simulink model "Isat"  (Simulink 7.5)
settings: Solver=ode45  StartTime=0.0  StopTime=10.0  RelTol=1e-3
settings Model: Creator=dell  LastModifiedBy=dell

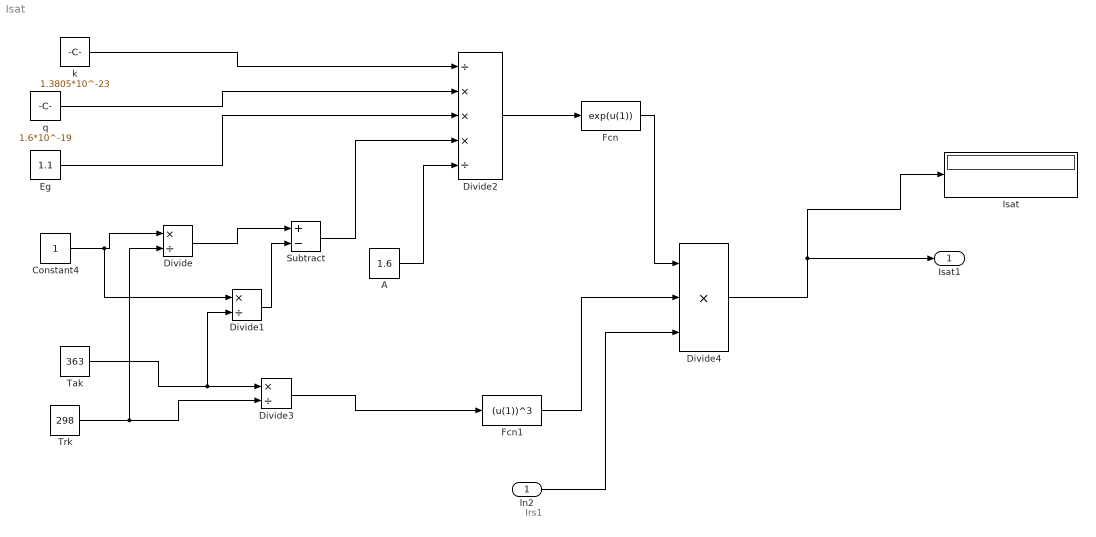
== system Isat ==
  note: Irs1
  In2 : Inport  OutDataType=fixdt(1, 16)  OutScaling=2^0
  A : Constant  Value=1.6  OutDataType=fixdt(1, 16)  OutScaling=2^0
  Constant4 : Constant  OutDataType=fixdt(1, 16)  OutScaling=2^0
  Divide : Product  Inputs=*/  OutDataType=fixdt(1, 16)  OutScaling=2^-10
  Divide1 : Product  Inputs=*/  OutDataType=fixdt(1, 16)  OutScaling=2^-10
  Divide2 : Product  Inputs=/***/  OutDataType=fixdt(1, 16)  OutScaling=2^-10
  Divide3 : Product  Inputs=*/  OutDataType=fixdt(1, 16)  OutScaling=2^-10
  Divide4 : Product  Inputs=***  OutDataType=fixdt(1, 16)  OutScaling=2^-10
  Eg : Constant  Value=1.1  OutDataType=fixdt(1, 16)  OutScaling=2^0
  Fcn : Fcn  Expr=exp(u(1))
  Fcn1 : Fcn  Expr=(u(1))^3
  Isat : Display
  Subtract : Sum  Inputs=+-  OutDataType=fixdt(1, 16)  OutScaling=2^-10
  Tak : Constant  Value=363  OutDataType=fixdt(1, 16)  OutScaling=2^0
  Trk : Constant  Value=298  OutDataType=fixdt(1, 16)  OutScaling=2^0
  k : Constant  Value=1.3805*10^-23  OutDataType=fixdt(1, 16)  OutScaling=2^0
  q : Constant  Value=1.6*10^-19  OutDataType=fixdt(1, 16)  OutScaling=2^0
  Isat1 : Outport  OutDataType=fixdt(1, 16)  OutScaling=2^0
  wires:
  k/1 -> Divide2/1
  q/1 -> Divide2/2
  Eg/1 -> Divide2/3
  Constant4/1 -> Divide/1, Divide1/1
  Tak/1 -> Divide3/1, Divide1/2
  Trk/1 -> Divide3/2, Divide/2
  Divide/1 -> Subtract/1
  Divide1/1 -> Subtract/2
  Subtract/1 -> Divide2/4
  A/1 -> Divide2/5
  Divide2/1 -> Fcn/1
  Divide4/1 -> Isat/1, Isat1/1
  Fcn/1 -> Divide4/1
  Divide3/1 -> Fcn1/1
  Fcn1/1 -> Divide4/2
  In2/1 -> Divide4/3
